simulink library "common_lib"  (R2023a)
settings: Solver=ode45  StartTime=0.0  StopTime=10.0  RelTol=1e-3
undefined symbols (not defined in the file): ACCEL_PRE_MULT, APDT_SrvcMgr_IRVHVDCSubFcnReq, C_C1GearNumbers, C_C1GearRatios, C_Calibration, C_DitherWaveform, C_GearOffset, C_GearRatioIn, C_GearRatioInverseOut, C_GearRatioOut, CLUTCH_INNER_LOOP_UPDATE_RATE, CONSTANT, DEGRADED_MODE_SIZE, Dem_EventStatusType, DiscIntNeverNeededParam, F_FAULT_ENUM, F_NOFAULT, F_OUTOFRANGE, F_RATELIMIT, FALSE, FMI14_SPECIAL_INSTRUCTIONS, FMI20_DATA_DRIFTED_HIGH, FMI21_DATA_DRIFTED_LOW, FMI29_RESERVED_FOR_SAE_ASSIGNMENT, FMI30_RESERVED_FOR_SAE_ASSIGNMENT, FMI31_CONDITION_EXISTS, FMI32_NO_FAULT, IC, k_accel, k_mean, MAX_UINT32, MEAN_PRE_MULT, NTriggers, QLTY_SIGNAL_FAILED, QLTY_SIGNAL_FULLY_FUNCTION, QLTY_SIGNAL_SUBSTITUTED_BY_1ST_CHOICE, QLTY_SIGNAL_SUBSTITUTED_BY_2ND_CHOICE, QLTY_SIGNAL_SUBSTITUTED_BY_3RD_CHOICE, QLTY_SIGNAL_SUBSTITUTED_BY_4TH_CHOICE, SAMPLE_TIME_100us, SAMPLETIME_10ms_Int, SATURATION_U16, simin, T_TestPoint, TF_FALSE, TF_TRUE, TimeStep, TRUE, WORKSPACE_UPDATE_RATE, ZERO, Zero
libraries: $bdroot x123, simulink x28, simulink_extras x4, MBD_EPS_Local_Blockset x4
(part 6 of 10)

== system common_lib/Diagnostics/DiagDbncCntrLite ==
  DiagFaultCntThresh : Inport
  DiagPassCntThresh : Inport  Port=2
  DiagFaultActive : Inport  Port=3
  DiagReset : Inport  Port=4
  diagHealEn : Inport  Port=5
  Constant1 : Constant  Value=int16(1)
  Constant2 : Constant  Value=int16(1)
  DiagDebounce_CCaller : CCaller  FunctionName=DiagDebounceLite  PortSpecificationStruct="%)30     .    :!    8    (     @         %    \"     D    !     0         %  0 \"0    $    _    07)G3F%M90  4&]R=$YA;64 4V-O<&4     26YD97@     5'EP90      4VEZ90      27-';&]B86P   X   !     !@    @    $          4    (     0   !     !         !     0    9&EA9T9A=6QT0V]U;G1E<@X   !     !@    @    $          4    (     0   !     !         !     0    9&EA9T9A=6QT0V]U;G1E<@X   !     !@    @    $     ...(+5283 chars)"
  Unit Delay : UnitDelay  SampleTime=-1  HasFrameUpgradeWarning=on
      settings: AttributesFormatString=%<InitialCondition>
  Unit Delay1 : UnitDelay  InitialCondition=int8(0)  SampleTime=-1  HasFrameUpgradeWarning=on
      settings: AttributesFormatString=%<InitialCondition>
  DiagCurrState : Outport  VectorParamsAs1DForOutWhenUnconnected=off
  wires:
  diagHealEn/1 -> DiagDebounce_CCaller/9
  Constant2/1 -> DiagDebounce_CCaller/8
  Constant1/1 -> DiagDebounce_CCaller/7
  DiagReset/1 -> DiagDebounce_CCaller/4
  DiagDebounce_CCaller/2 -> DiagCurrState/1, Unit Delay1/1
  DiagPassCntThresh/1 -> DiagDebounce_CCaller/6
  DiagFaultCntThresh/1 -> DiagDebounce_CCaller/5
  DiagFaultActive/1 -> DiagDebounce_CCaller/3
  Unit Delay/1 -> DiagDebounce_CCaller/1
  Unit Delay1/1 -> DiagDebounce_CCaller/2
  DiagDebounce_CCaller/1 -> Unit Delay/1

== system common_lib/Diagnostics/DiagFaultCounter ==
  diagFaultActive : Inport
  diagStartUpComp : Inport  Port=2
  diagReset : Inport  Port=3
  diagEnable : Inport  Port=4
  diagDbncEnab : Inport  Port=5
  diagFaultCntThresh : Inport  Port=6
  diagPassCntThresh : Inport  Port=7
  diagUpCnt : Inport  Port=8
  diagDnCnt : Inport  Port=9
  diagHealEn : Inport  Port=10
  DiagFaulCounter : Stateflow chart  TreatAsAtomicUnit=on
  diagFaultStatus : Outport  OutputWhenDisabled=reset  InitialOutput=Dem_EventStatusType.DEM_EVENT_STATUS_INIT  VectorParamsAs1DForOutWhenUnconnected=off
  wires:
  diagHealEn/1 -> DiagFaulCounter/10(diagHealEn)
  diagPassCntThresh/1 -> DiagFaulCounter/7(diagPassCntThresh)
  diagStartUpComp/1 -> DiagFaulCounter/2(diagStartUpComp)
  diagDbncEnab/1 -> DiagFaulCounter/5(diagDbncEnab)
  DiagFaulCounter/1(diagFaultStatus) -> diagFaultStatus/1
  diagEnable/1 -> DiagFaulCounter/4(diagEnable)
  diagDnCnt/1 -> DiagFaulCounter/9(diagDnCnt)
  diagUpCnt/1 -> DiagFaulCounter/8(diagUpCnt)
  diagReset/1 -> DiagFaulCounter/3(diagReset)
  diagFaultCntThresh/1 -> DiagFaulCounter/6(diagFaultCntThresh)
  diagFaultActive/1 -> DiagFaulCounter/1(diagFaultActive)

== system common_lib/Diagnostics/ExtractValue ==
  in : Inport  OutDataTypeStr=Bus: BO_InputSignal
  Bus Selector : BusSelector  OutputSignals=value,FMI
  value : Outport  VectorParamsAs1DForOutWhenUnconnected=off
  FMI : Outport  Port=2  VectorParamsAs1DForOutWhenUnconnected=off
  wires:
  Bus Selector/2 -> FMI/1  "<FMI>"
  in/1 -> Bus Selector/1
  Bus Selector/1 -> value/1  "<value>"

== system common_lib/Diagnostics/FMIUpdate ==
  UpdateFaultStatus : Inport
  FMI_In : Inport  Port=2
  FMI_UpdateValue : Inport  Port=3
  Constant2 : Constant  Value=FMI32_NO_FAULT  SampleTime=-1
  Relational Operator3 : RelationalOperator  Operator=~=  ZeroCross=off  InputSameDT=off
  Switch : Switch  Threshold=0.5  ZeroCross=off  SaturateOnIntegerOverflow=off  InputSameDT=off
  Switch1 : Switch  Threshold=0.5  ZeroCross=off  SaturateOnIntegerOverflow=off  InputSameDT=off
  FMI_Out : Outport  VectorParamsAs1DForOutWhenUnconnected=off
  wires:
  Switch1/1 -> FMI_Out/1
  FMI_In/1 -> Switch/3, Switch1/1, Relational Operator3/1
  Relational Operator3/1 -> Switch1/2
  Switch/1 -> Switch1/3
  FMI_UpdateValue/1 -> Switch/1
  UpdateFaultStatus/1 -> Switch/2
  Constant2/1 -> Relational Operator3/2

== system common_lib/Diagnostics/Fault Debounce Lv1 Boolean Input ==
  diagInput : Inport
  diagStartUpComp : Inport  Port=2
  diagUpCnt : Inport  Port=3
  diagDnCnt : Inport  Port=4
  diagFaultCntThresh : Inport  Port=5
  diagPassCntThresh : Inport  Port=6
  diagDbncEnab : Inport  Port=7
  diagReset : Inport  Port=8
  diagEnable : Inport  Port=9
  diagHealEn : Inport  Port=10
  diagPreestorageEn : Inport  Port=11
  diagJumpDownEn : Inport  Port=12
  Ccaller_DiagLv1 : $bdroot/Diagnostics/Ccaller_DiagLv1  SystemSampleTime=-1  VariantActivationTime=update diagram  Latency=0  AutoFrameSizeCalculation=off
  diagFaultStatus : Outport  OutputWhenDisabled=reset  InitialOutput=Dem_EventStatusType.DEM_EVENT_STATUS_INIT  VectorParamsAs1DForOutWhenUnconnected=off
  diagPreestorageTrigger : Outport  Port=2  OutputWhenDisabled=reset  InitialOutput=Dem_EventStatusType.DEM_EVENT_STATUS_INIT  VectorParamsAs1DForOutWhenUnconnected=off
  wires:
  diagStartUpComp/1 -> Ccaller_DiagLv1/2
  diagReset/1 -> Ccaller_DiagLv1/3
  diagEnable/1 -> Ccaller_DiagLv1/4
  diagDbncEnab/1 -> Ccaller_DiagLv1/5
  diagFaultCntThresh/1 -> Ccaller_DiagLv1/6
  diagPassCntThresh/1 -> Ccaller_DiagLv1/7
  diagUpCnt/1 -> Ccaller_DiagLv1/8
  diagDnCnt/1 -> Ccaller_DiagLv1/9
  diagHealEn/1 -> Ccaller_DiagLv1/10
  diagPreestorageEn/1 -> Ccaller_DiagLv1/11
  diagJumpDownEn/1 -> Ccaller_DiagLv1/12
  Ccaller_DiagLv1/2 -> diagPreestorageTrigger/1
  Ccaller_DiagLv1/1 -> diagFaultStatus/1
  diagInput/1 -> Ccaller_DiagLv1/1

== system common_lib/Diagnostics/Fault Debounce Lv1 state Input ==
  diagInput : Inport
  diagStartUpComp : Inport  Port=2
  diagMaxVal : Inport  Port=3
  diagMinVal : Inport  Port=4
  diagUpCnt : Inport  Port=5
  diagDnCnt : Inport  Port=6
  diagFaultCntThresh : Inport  Port=7
  diagPassCntThresh : Inport  Port=8
  diagDbncEnab : Inport  Port=9
  diagReset : Inport  Port=10
  diagEnable : Inport  Port=11
  diagHealEn : Inport  Port=12
  diagPreestorageEn : Inport  Port=13
  diagJumpDownEn : Inport  Port=14
  Ccaller_DiagLv1 : $bdroot/Diagnostics/Ccaller_DiagLv1  SystemSampleTime=-1  VariantActivationTime=update diagram  Latency=0  AutoFrameSizeCalculation=off
  OR : Logic  Operator=OR  AllPortsSameDT=off  OutDataTypeStr=boolean
  Relational Operator : RelationalOperator  OutDataTypeStr=boolean  ZeroCross=off  InputSameDT=off
  Relational Operator1 : RelationalOperator  Operator=<=  OutDataTypeStr=boolean  ZeroCross=off  InputSameDT=off
  diagFaultStatus : Outport  OutputWhenDisabled=reset  InitialOutput=Dem_EventStatusType.DEM_EVENT_STATUS_INIT  VectorParamsAs1DForOutWhenUnconnected=off
  diagPreestorageTrigger : Outport  Port=2  OutputWhenDisabled=reset  InitialOutput=Dem_EventStatusType.DEM_EVENT_STATUS_INIT  VectorParamsAs1DForOutWhenUnconnected=off
  wires:
  diagMaxVal/1 -> Relational Operator/2
  diagReset/1 -> Ccaller_DiagLv1/3
  diagDnCnt/1 -> Ccaller_DiagLv1/9
  diagFaultCntThresh/1 -> Ccaller_DiagLv1/6
  diagPassCntThresh/1 -> Ccaller_DiagLv1/7
  diagUpCnt/1 -> Ccaller_DiagLv1/8
  Relational Operator/1 -> OR/1
  diagStartUpComp/1 -> Ccaller_DiagLv1/2
  diagDbncEnab/1 -> Ccaller_DiagLv1/5
  diagInput/1 -> Relational Operator/1, Relational Operator1/1
  diagHealEn/1 -> Ccaller_DiagLv1/10
  diagMinVal/1 -> Relational Operator1/2
  OR/1 -> Ccaller_DiagLv1/1
  Relational Operator1/1 -> OR/2
  diagEnable/1 -> Ccaller_DiagLv1/4
  diagPreestorageEn/1 -> Ccaller_DiagLv1/11
  diagJumpDownEn/1 -> Ccaller_DiagLv1/12
  Ccaller_DiagLv1/1 -> diagFaultStatus/1
  Ccaller_DiagLv1/2 -> diagPreestorageTrigger/1

== system common_lib/Diagnostics/FaultStatusUpdate ==
  FMI_In : Inport
  DriftLow : Inport  Port=2
  DriftHigh : Inport  Port=3
  SpecialInstructions : Inport  Port=4
  ConditionExists : Inport  Port=5
  DriftLowSubReqest : Inport  Port=6
  DriftLowSubReqest1 : Inport  Port=7
  Constant : Constant  Value=FMI14_SPECIAL_INSTRUCTIONS  SampleTime=-1
  Constant1 : Constant  Value=FMI21_DATA_DRIFTED_LOW  SampleTime=-1
  Constant2 : Constant  Value=FMI20_DATA_DRIFTED_HIGH  SampleTime=-1
  Constant3 : Constant  Value=FMI29_RESERVED_FOR_SAE_ASSIGNMENT  SampleTime=-1
  Constant4 : Constant  Value=FMI32_NO_FAULT  SampleTime=-1
  Constant5 : Constant  Value=FMI30_RESERVED_FOR_SAE_ASSIGNMENT  SampleTime=-1
  Constant6 : Constant  Value=FMI31_CONDITION_EXISTS  SampleTime=-1
  Relational Operator3 : RelationalOperator  Operator=~=  ZeroCross=off  InputSameDT=off
  Switch{,1..6} (7 alike) : Switch  Threshold=0.5  ZeroCross=off  SaturateOnIntegerOverflow=off  InputSameDT=off
  FMI_Out : Outport  VectorParamsAs1DForOutWhenUnconnected=off
  wires:
  Switch1/1 -> FMI_Out/1
  Constant4/1 -> Relational Operator3/2
  Switch/1 -> Switch1/3
  Relational Operator3/1 -> Switch1/2
  FMI_In/1 -> Relational Operator3/1, Switch1/1, Switch6/3
  Switch2/1 -> Switch/3
  Switch3/1 -> Switch2/3
  Switch4/1 -> Switch3/3
  DriftLow/1 -> Switch/2
  Constant1/1 -> Switch/1
  Constant2/1 -> Switch2/1
  DriftHigh/1 -> Switch2/2
  Constant/1 -> Switch3/1
  SpecialInstructions/1 -> Switch3/2
  Constant6/1 -> Switch4/1
  ConditionExists/1 -> Switch4/2
  Constant3/1 -> Switch5/1
  DriftLowSubReqest/1 -> Switch5/2
  Constant5/1 -> Switch6/1
  DriftLowSubReqest1/1 -> Switch6/2
  Switch6/1 -> Switch5/3
  Switch5/1 -> Switch4/3

== system common_lib/Diagnostics/Heal Enable Cnt With Reset ==
  Diag_FltSts : Inport
  Mode_Req : Inport  Port=2
  Diag_TogLim_C : Inport  Port=3
  Accumulator : UnitDelay  SampleTime=-1  HasFrameUpgradeWarning=on
      settings: AttributesFormatString=ic=%<X0>
  ActFltSts : RelationalOperator  Operator===  ZeroCross=off  InputSameDT=off
  CntrCnd : Switch  Criteria=u2 ~= 0  Threshold=0.5  ZeroCross=off  SaturateOnIntegerOverflow=off  InputSameDT=off
      settings: AttributesFormatString=%<Criteria>
  DIAG_FLTD : Constant  OutDataTypeStr=uint8  SampleTime=-1
  DIAG_FLTD1 : Constant  OutDataTypeStr=uint8  SampleTime=-1
  EdgeDetection : Logic  AllPortsSameDT=off
  HealEnaCnd : RelationalOperator  Operator=<=  OutDataTypeStr=boolean  ZeroCross=off  InputSameDT=off
  HealEnaCnd_Old : UnitDelay  SampleTime=-1  HasFrameUpgradeWarning=on
      settings: AttributesFormatString=ic=%<X0>
  IncrCond : Logic  AllPortsSameDT=off
  OldFltSts : RelationalOperator  Operator=~=  ZeroCross=off  InputSameDT=off
  PM_STANDBY : Constant  Value=0  OutDataTypeStr=uint8  SampleTime=-1
  Plus_One : Constant  OutDataTypeStr=uint8  SampleTime=-1
  Plus_Zero : Constant  Value=0  OutDataTypeStr=uint8  SampleTime=-1
  ResetCond : RelationalOperator  Operator===  ZeroCross=off  InputSameDT=off
  Reset_Value : Constant  Value=0  OutDataTypeStr=uint8  SampleTime=-1
  RstCnd : Switch  Criteria=u2 ~= 0  Threshold=0.5  ZeroCross=off  SaturateOnIntegerOverflow=off  InputSameDT=off
      settings: AttributesFormatString=%<Criteria>
  Sum2 : Sum  Inputs=|++
  Unit Delay1 : UnitDelay  InitialCondition=FALSE  SampleTime=-1  HasFrameUpgradeWarning=on
      settings: AttributesFormatString=ic=%<X0>
  Diag_HealEna : Outport  VectorParamsAs1DForOutWhenUnconnected=off
  wires:
  RstCnd/1 -> Accumulator/1, HealEnaCnd/1
  Sum2/1 -> RstCnd/3
  ResetCond/1 -> RstCnd/2
  Diag_TogLim_C/1 -> HealEnaCnd/2
  Plus_Zero/1 -> CntrCnd/3
  OldFltSts/1 -> EdgeDetection/2
  Unit Delay1/1 -> OldFltSts/1
  HealEnaCnd_Old/1 -> IncrCond/2
  HealEnaCnd/1 -> Diag_HealEna/1, HealEnaCnd_Old/1
  Plus_One/1 -> CntrCnd/1
  CntrCnd/1 -> Sum2/1
  IncrCond/1 -> CntrCnd/2
  Diag_FltSts/1 -> Unit Delay1/1, ActFltSts/1
  Reset_Value/1 -> RstCnd/1
  ActFltSts/1 -> EdgeDetection/1
  DIAG_FLTD1/1 -> OldFltSts/2
  DIAG_FLTD/1 -> ActFltSts/2
  Accumulator/1 -> Sum2/2
  Mode_Req/1 -> ResetCond/1
  PM_STANDBY/1 -> ResetCond/2
  EdgeDetection/1 -> IncrCond/1

== system common_lib/Diagnostics/KeepAlive ==
  State : Inport  OutDataTypeStr=boolean  PortDimensions=1
  A : Inport  Port=2  PortDimensions=1
  B : Inport  Port=3  PortDimensions=1
  Delay : UnitDelay  InitialCondition=false  SampleTime=-1  HasFrameUpgradeWarning=on
  Logical Operator : Logic  Operator=OR  AllPortsSameDT=off  OutDataTypeStr=boolean
  RelOp : RelationalOperator  Operator===  OutDataTypeStr=boolean
  Enable : Outport  OutDataTypeStr=boolean  PortDimensions=1  VectorParamsAs1DForOutWhenUnconnected=off
  Rel : Outport  Port=2  OutDataTypeStr=boolean  PortDimensions=1  VectorParamsAs1DForOutWhenUnconnected=off
  wires:
  RelOp/1 -> Logical Operator/2, Rel/1
  Logical Operator/1 -> Enable/1
  B/1 -> RelOp/2
  Delay/1 -> Logical Operator/1
  State/1 -> Delay/1
  A/1 -> RelOp/1

== system common_lib/Diagnostics/LogicBasedActivation ==
  note: Logic Based Activation
  Enable : Inport  OutDataTypeStr=boolean  PortDimensions=1
  DMToAdd : Inport  Port=2  OutDataTypeStr=uint32  PortDimensions=DM_SIZE
  Add : Inport  Port=3  OutDataTypeStr=boolean  PortDimensions=1
  DMPackedData_in : Inport  Port=4  OutDataTypeStr=uint32  PortDimensions=DM_SIZE
  Bitwise Operator : simulink/Logic and Bit Operations/Bitwise Operator  logicop=OR  UseBitMask=off  NumInputPorts=2  BitMask=bin2dec('11011001')  BitMaskRealWorld=Stored Integer
  Logical Operator1 : Logic  AllPortsSameDT=off
  Switch3 : Switch  Threshold=0.5  ZeroCross=off  SaturateOnIntegerOverflow=off  InputSameDT=off
  DMPackedData_out : Outport  OutDataTypeStr=uint32  PortDimensions=DM_SIZE  VectorParamsAs1DForOutWhenUnconnected=off
  wires:
  Switch3/1 -> DMPackedData_out/1
  Bitwise Operator/1 -> Switch3/1
  DMToAdd/1 -> Bitwise Operator/1
  DMPackedData_in/1 -> Bitwise Operator/2, Switch3/3
  Logical Operator1/1 -> Switch3/2
  Enable/1 -> Logical Operator1/1
  Add/1 -> Logical Operator1/2

== system common_lib/Diagnostics/LogicBasedDeactivation ==
  note: Logic Based Deactivation
  Enable : Inport  OutDataTypeStr=boolean  PortDimensions=1
  DMToRemove : Inport  Port=2  OutDataTypeStr=uint32  PortDimensions=DM_SIZE
  Remove : Inport  Port=3  OutDataTypeStr=boolean  PortDimensions=1
  DMPackedData_in : Inport  Port=4  OutDataTypeStr=uint32  PortDimensions=DM_SIZE
  Bitwise Operator : simulink/Logic and Bit Operations/Bitwise Operator  logicop=AND  UseBitMask=off  NumInputPorts=2  BitMask=bin2dec('11011001')  BitMaskRealWorld=Stored Integer
  Bitwise Operator1 : simulink/Logic and Bit Operations/Bitwise Operator  logicop=NOT  UseBitMask=off  BitMask=bin2dec('11011001')  BitMaskRealWorld=Stored Integer
  Logical Operator1 : Logic  AllPortsSameDT=off
  Switch3 : Switch  Threshold=0.5  ZeroCross=off  SaturateOnIntegerOverflow=off  InputSameDT=off
  DMPackedData_out : Outport  OutDataTypeStr=uint32  PortDimensions=DM_SIZE  VectorParamsAs1DForOutWhenUnconnected=off
  wires:
  Remove/1 -> Logical Operator1/2
  Enable/1 -> Logical Operator1/1
  Logical Operator1/1 -> Switch3/2
  DMPackedData_in/1 -> Switch3/3, Bitwise Operator/2
  DMToRemove/1 -> Bitwise Operator1/1
  Bitwise Operator/1 -> Switch3/1
  Switch3/1 -> DMPackedData_out/1
  Bitwise Operator1/1 -> Bitwise Operator/1

== system common_lib/Diagnostics/OOR Fault Detect Enum ==
  note: Common Library::Diagnostics::Out of Range Fault Detection with Enable for Enum
  in : Inport
  Enable : Inport  Port=2
  Logical Operator1 : Logic  Operator=NOT  AllPortsSameDT=off  OutDataTypeStr=boolean
  Switch : Switch  Criteria=u2 ~= 0  InputSameDT=off
  detect fault : Subsystem
  false1 : Constant  Value=FALSE  OutDataTypeStr=boolean
  out : Outport  VectorParamsAs1DForOutWhenUnconnected=off
  fault? : Outport  Port=2  VectorParamsAs1DForOutWhenUnconnected=off
  wires:
  Enable/1 -> Logical Operator1/1, detect fault/Enable
  Switch/1 -> fault?/1
  false1/1 -> Switch/1
  detect fault/1(fault set) -> Switch/3
  in/1 -> out/1, detect fault/1(In1)
  Logical Operator1/1 -> Switch/2

== system common_lib/Diagnostics/OOR Fault Detection ==
  note: Common Library::Diagnostics::Out of Range Fault Detection with Enable
  in : Inport
  Enable : Inport  Port=2
  Logical Operator3 : Logic  Operator=NOT  AllPortsSameDT=off  OutDataTypeStr=boolean
  Switch : Switch  Criteria=u2 ~= 0  InputSameDT=off
  detect fault : Subsystem
  false : Constant  Value=FALSE  OutDataTypeStr=boolean
  out : Outport  VectorParamsAs1DForOutWhenUnconnected=off
  fault? : Outport  Port=2  VectorParamsAs1DForOutWhenUnconnected=off
  wires:
  in/1 -> out/1, detect fault/1(In1)
  Logical Operator3/1 -> Switch/2
  detect fault/1(fault set) -> Switch/3
  false/1 -> Switch/1
  Switch/1 -> fault?/1
  Enable/1 -> Logical Operator3/1, detect fault/Enable

== system common_lib/Diagnostics/SetFMI ==
  FMI_in : Inport  OutDataTypeStr=uint8  PortDimensions=1
  Active1 : Inport  Port=2  OutDataTypeStr=boolean  PortDimensions=1
  Active2 : Inport  Port=3  OutDataTypeStr=boolean  PortDimensions=1
  Active3 : Inport  Port=4  OutDataTypeStr=boolean  PortDimensions=1
  Active4 : Inport  Port=5  OutDataTypeStr=boolean  PortDimensions=1
  Active5 : Inport  Port=6  OutDataTypeStr=boolean  PortDimensions=1
  Active6 : Inport  Port=7  OutDataTypeStr=boolean  PortDimensions=1
  Active7 : Inport  Port=8  OutDataTypeStr=boolean  PortDimensions=1
  Constant : Constant  Value=PRIORITY_1_FMI
  Constant1 : Constant  Value=PRIORITY_2_FMI
  Constant2 : Constant  Value=PRIORITY_3_FMI
  Constant3 : Constant  Value=PRIORITY_4_FMI
  Constant4 : Constant  Value=PRIORITY_5_FMI
  Constant5 : Constant  Value=PRIORITY_6_FMI
  Constant6 : Constant  Value=PRIORITY_7_FMI
  IF_ELSE_LADDER : Subsystem  TreatAsAtomicUnit=on
      settings: RTWSystemCode=Inline
  FMI_out : Outport  VectorParamsAs1DForOutWhenUnconnected=off
  wires:
  IF_ELSE_LADDER/1(FMI_out) -> FMI_out/1
  Active7/1 -> IF_ELSE_LADDER/8(Active7)
  Active6/1 -> IF_ELSE_LADDER/7(Active6)
  Active5/1 -> IF_ELSE_LADDER/6(Active5)
  Active4/1 -> IF_ELSE_LADDER/5(Active4)
  Active3/1 -> IF_ELSE_LADDER/4(Active3)
  Active2/1 -> IF_ELSE_LADDER/3(Active2)
  Active1/1 -> IF_ELSE_LADDER/2(Active1)
  FMI_in/1 -> IF_ELSE_LADDER/1(FMI_in)
  Constant6/1 -> IF_ELSE_LADDER/15(FMI_7)
  Constant5/1 -> IF_ELSE_LADDER/14(FMI_6)
  Constant4/1 -> IF_ELSE_LADDER/13(FMI_5)
  Constant3/1 -> IF_ELSE_LADDER/12(FMI_4)
  Constant2/1 -> IF_ELSE_LADDER/11(FMI_3)
  Constant1/1 -> IF_ELSE_LADDER/10(FMI_2)
  Constant/1 -> IF_ELSE_LADDER/9(FMI_1)

== system common_lib/Diagnostics/SignalSubstitution ==
  Signal_in : Inport  OutDataTypeStr=single  PortDimensions=1
  SignalFaulted : Inport  Port=2  OutDataTypeStr=boolean  PortDimensions=1
  FirstChoiceSubstitute : Inport  Port=3  OutDataTypeStr=single  PortDimensions=1
  FirstChoiceFaulted : Inport  Port=4  OutDataTypeStr=boolean  PortDimensions=1
  SecondChoiceSubstitute : Inport  Port=5  OutDataTypeStr=single  PortDimensions=1
  SecondChoiceFaulted : Inport  Port=6  OutDataTypeStr=boolean  PortDimensions=1
  ThirdChoiceSubstitute : Inport  Port=7  OutDataTypeStr=single  PortDimensions=1
  ThirdChoiceFaulted : Inport  Port=8  OutDataTypeStr=boolean  PortDimensions=1
  FourthChoiceSubstitute : Inport  Port=9  OutDataTypeStr=single  PortDimensions=1
  FourthChoiceFaulted : Inport  Port=10  OutDataTypeStr=boolean  PortDimensions=1
  FailedValue : Inport  Port=11  OutDataTypeStr=single  PortDimensions=1
  If : If  NumInputs=5  IfExpression=~u1  ElseIfExpressions=~u2, ~u3, ~u4, ~u5
  If Action Subsystem : Subsystem  TreatAsAtomicUnit=on
  If Action Subsystem1 : Subsystem  TreatAsAtomicUnit=on
  If Action Subsystem2 : Subsystem  TreatAsAtomicUnit=on
  If Action Subsystem3 : Subsystem  TreatAsAtomicUnit=on
  If Action Subsystem4 : Subsystem  TreatAsAtomicUnit=on
  If Action Subsystem5 : Subsystem  TreatAsAtomicUnit=on
  Merge : Merge  Inputs=6
  Merge1 : Merge  Inputs=6
  Signal_out : Outport  OutDataTypeStr=single  PortDimensions=1  VectorParamsAs1DForOutWhenUnconnected=off
  Qlty : Outport  Port=2  OutDataTypeStr=uint8  PortDimensions=1  VectorParamsAs1DForOutWhenUnconnected=off
  wires:
  If Action Subsystem2/2(Qlty) -> Merge1/3
  If Action Subsystem2/1(Signal) -> Merge/3
  If Action Subsystem1/2(Qlty) -> Merge1/2
  If Action Subsystem3/1(Signal) -> Merge/4
  Merge/1 -> Signal_out/1
  If Action Subsystem4/2(Qlty) -> Merge1/5
  If Action Subsystem/1(Signal) -> Merge/1
  If Action Subsystem4/1(Signal) -> Merge/5
  If Action Subsystem5/1(Signal) -> Merge/6
  If Action Subsystem1/1(Signal) -> Merge/2
  If Action Subsystem3/2(Qlty) -> Merge1/4
  If Action Subsystem/2(Qlty) -> Merge1/1
  If Action Subsystem5/2(Qlty) -> Merge1/6
  Merge1/1 -> Qlty/1
  If/3 -> If Action Subsystem2/Action
  Signal_in/1 -> If Action Subsystem/1(NoSubstitute)
  SecondChoiceSubstitute/1 -> If Action Subsystem2/1(SecondChoice)
  If/1 -> If Action Subsystem/Action
  FirstChoiceFaulted/1 -> If/2
  If/2 -> If Action Subsystem1/Action
  SecondChoiceFaulted/1 -> If/3
  FourthChoiceFaulted/1 -> If/5
  FirstChoiceSubstitute/1 -> If Action Subsystem1/1(FirstChoice)
  If/4 -> If Action Subsystem3/Action
  ThirdChoiceFaulted/1 -> If/4
  FailedValue/1 -> If Action Subsystem5/1(FailedValue)
  If/5 -> If Action Subsystem4/Action
  If/6 -> If Action Subsystem5/Action
  SignalFaulted/1 -> If/1
  FourthChoiceSubstitute/1 -> If Action Subsystem4/1(FourthChoice)
  ThirdChoiceSubstitute/1 -> If Action Subsystem3/1(ThirdChoice)

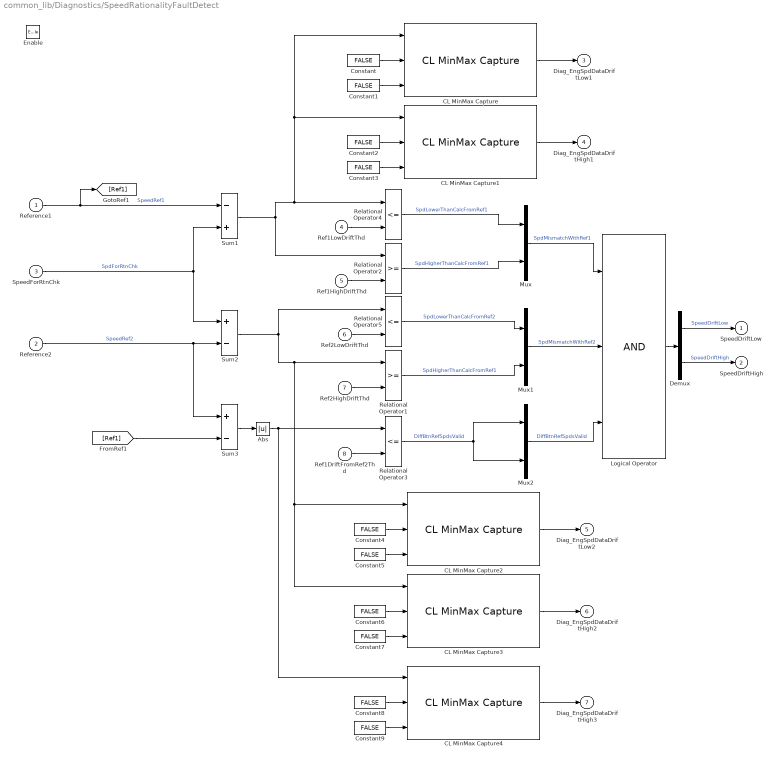
== system common_lib/Diagnostics/SpeedRationalityFaultDetect ==
  Reference1 : Inport
  Reference2 : Inport  Port=2
  SpeedForRtnChk : Inport  Port=3
  Ref1LowDriftThd : Inport  Port=4
  Ref1HighDriftThd : Inport  Port=5
  Ref2LowDriftThd : Inport  Port=6
  Ref2HighDriftThd : Inport  Port=7
  Ref1DriftFromRef2Thd : Inport  Port=8
  Enable : EnablePort  ZeroCross=off
  Abs : Abs  ZeroCross=off  SaturateOnIntegerOverflow=off
  CL MinMax Capture : $bdroot/Diag/CL MinMax Capture  CaptureType=Min  InDataType=single
  CL MinMax Capture1 : $bdroot/Diag/CL MinMax Capture  CaptureType=Max  InDataType=single
  CL MinMax Capture2 : $bdroot/Diag/CL MinMax Capture  CaptureType=Min  InDataType=single
  CL MinMax Capture3 : $bdroot/Diag/CL MinMax Capture  CaptureType=Max  InDataType=single
  CL MinMax Capture4 : $bdroot/Diag/CL MinMax Capture  CaptureType=Max  InDataType=single
  Constant{,1..9} (10 alike) : Constant  Value=FALSE  SampleTime=-1
  Demux : Demux  Outputs=2
  Logical Operator : Logic  Inputs=3  AllPortsSameDT=off
  Mux : Mux  Inputs=2
  Mux1 : Mux  Inputs=2
  Mux2 : Mux  Inputs=2
  Relational Operator1 : RelationalOperator  ZeroCross=off  InputSameDT=off
  Relational Operator2 : RelationalOperator  ZeroCross=off  InputSameDT=off
  Relational Operator3 : RelationalOperator  Operator=<=  ZeroCross=off  InputSameDT=off
  Relational Operator4 : RelationalOperator  Operator=<=  ZeroCross=off  InputSameDT=off
  Relational Operator5 : RelationalOperator  Operator=<=  ZeroCross=off  InputSameDT=off
  Sum1 : Sum  Inputs=-+
  Sum2 : Sum  Inputs=+-
  Sum3 : Sum  Inputs=+-
  SpeedDriftLow : Outport  OutputWhenDisabled=reset  InitialOutput=[0]  VectorParamsAs1DForOutWhenUnconnected=off
  SpeedDriftHigh : Outport  Port=2  OutputWhenDisabled=reset  InitialOutput=[0]  VectorParamsAs1DForOutWhenUnconnected=off
  Diag_EngSpdDataDriftLow1 : Outport  Port=3  InitialOutput=[0]  VectorParamsAs1DForOutWhenUnconnected=off
  Diag_EngSpdDataDriftHigh1 : Outport  Port=4  InitialOutput=[0]  VectorParamsAs1DForOutWhenUnconnected=off
  Diag_EngSpdDataDriftLow2 : Outport  Port=5  InitialOutput=[0]  VectorParamsAs1DForOutWhenUnconnected=off
  Diag_EngSpdDataDriftHigh2 : Outport  Port=6  InitialOutput=[0]  VectorParamsAs1DForOutWhenUnconnected=off
  Diag_EngSpdDataDriftHigh3 : Outport  Port=7  InitialOutput=[0]  VectorParamsAs1DForOutWhenUnconnected=off
  wires:
  Constant9/1 -> CL MinMax Capture4/3
  Constant8/1 -> CL MinMax Capture4/2
  CL MinMax Capture4/1 -> Diag_EngSpdDataDriftHigh3/1
  CL MinMax Capture3/1 -> Diag_EngSpdDataDriftHigh2/1
  CL MinMax Capture2/1 -> Diag_EngSpdDataDriftLow2/1
  Constant7/1 -> CL MinMax Capture3/3
  Constant6/1 -> CL MinMax Capture3/2
  Constant5/1 -> CL MinMax Capture2/3
  Constant4/1 -> CL MinMax Capture2/2
  CL MinMax Capture1/1 -> Diag_EngSpdDataDriftHigh1/1
  CL MinMax Capture/1 -> Diag_EngSpdDataDriftLow1/1
  Constant3/1 -> CL MinMax Capture1/3
  Constant2/1 -> CL MinMax Capture1/2
  Constant1/1 -> CL MinMax Capture/3
  Constant/1 -> CL MinMax Capture/2
  Reference2/1 -> Sum3/1, Sum2/2  "SpeedRef2"
  Reference1/1 -> [Ref1], Sum1/1  "SpeedRef1"
  Ref2HighDriftThd/1 -> Relational Operator1/2
  Ref1HighDriftThd/1 -> Relational Operator2/2
  Logical Operator/1 -> Demux/1
  Demux/2 -> SpeedDriftHigh/1  "SpeedDriftHigh"
  Demux/1 -> SpeedDriftLow/1  "SpeedDriftLow"
  Mux2/1 -> Logical Operator/3  "DiffBtnRefSpdsValid"
  Mux1/1 -> Logical Operator/2  "SpdMismatchWithRef2"
  Mux/1 -> Logical Operator/1  "SpdMismatchWithRef1"
  Relational Operator1/1 -> Mux1/2  "SpdHigherThanCalcFromRef1"
  Relational Operator5/1 -> Mux1/1  "SpdLowerThanCalcFromRef2"
  Relational Operator4/1 -> Mux/1  "SpdLowerThanCalcFromRef1"
  Sum3/1 -> Abs/1
  Ref2LowDriftThd/1 -> Relational Operator5/2
  Ref1LowDriftThd/1 -> Relational Operator4/2
  Ref1DriftFromRef2Thd/1 -> Relational Operator3/2
  Abs/1 -> CL MinMax Capture4/1, Relational Operator3/1
  Sum2/1 -> Relational Operator5/1, Relational Operator1/1, CL MinMax Capture3/1, CL MinMax Capture2/1
  [Ref1] -> Sum3/2
  SpeedForRtnChk/1 -> Sum2/1, Sum1/2  "SpdForRtnChk"
  Relational Operator2/1 -> Mux/2  "SpdHigherThanCalcFromRef1"
  Sum1/1 -> Relational Operator2/1, Relational Operator4/1, CL MinMax Capture/1, CL MinMax Capture1/1
  Relational Operator3/1 -> Mux2/2, Mux2/1  "DiffBtnRefSpdsValid"

== system common_lib/Diagnostics/ToRWSignal ==
  in : Inport
  FMI : Inport  Port=2
  Bus Creator2 : BusCreator  Inputs=2  OutDataTypeStr=Bus: BO_InputSignal
  Data Type Conversion1 : DataTypeConversion  OutDataTypeStr=single  SaturateOnIntegerOverflow=off  RndMeth=Floor
  Data Type Conversion2 : DataTypeConversion  OutDataTypeStr=uint8  SaturateOnIntegerOverflow=off  RndMeth=Floor
  out : Outport  VectorParamsAs1DForOutWhenUnconnected=off
  wires:
  FMI/1 -> Data Type Conversion2/1
  Data Type Conversion2/1 -> Bus Creator2/2  "FMI"
  Data Type Conversion1/1 -> Bus Creator2/1  "value"
  in/1 -> Data Type Conversion1/1
  Bus Creator2/1 -> out/1

== system common_lib/Documentation/EatonLogo ==

== system common_lib/Documentation/LegalNoticeEaton ==

== system common_lib/Documentation/RequirementLinks ==
  DocBlock : simulink/Model-Wide Utilities/DocBlock  DocumentType=Text
      content=|
      | REQ_1234

== system common_lib/Documentation/SubsystemPath ==

== system common_lib/Fltrs/Fltr ==
  note: Common Library::Filters::Filter
  input : Inport
  tau : Inport  Port=2
  Constant : Constant  Value=single(0)  SampleTime=-1
  Constant1 : Constant  Value=false  SampleTime=-1
  Constant2 : Constant  Value=false  SampleTime=-1
  Data Type Conversion : DataTypeConversion  OutDataTypeStr=single  SaturateOnIntegerOverflow=off  RndMeth=Floor
  Data Type Conversion1 : DataTypeConversion  OutDataTypeStr=single  SaturateOnIntegerOverflow=off  RndMeth=Floor
  FilterCoreLogic1 : $bdroot/Fltrs/Fltr_wRO/FilterCoreLogic  SystemSampleTime=-1  VariantActivationTime=update diagram  Latency=0  AutoFrameSizeCalculation=off
  Signal Conversion : SignalConversion  ConversionOutput=Contiguous copy  OverrideOpt=on
  output : Outport  VectorParamsAs1DForOutWhenUnconnected=off
  wires:
  input/1 -> Data Type Conversion/1
  tau/1 -> Data Type Conversion1/1
  Signal Conversion/1 -> output/1
  FilterCoreLogic1/1 -> Signal Conversion/1
  Constant/1 -> FilterCoreLogic1/3
  Constant1/1 -> FilterCoreLogic1/4
  Constant2/1 -> FilterCoreLogic1/5
  Data Type Conversion/1 -> FilterCoreLogic1/1
  Data Type Conversion1/1 -> FilterCoreLogic1/2

== system common_lib/Fltrs/Fltr_wR ==
  note: Common Library::Filters::Filter with Reset
  note: This is a simple 1st order filter block with reset.
      |
      |     if reset is true (1) then output=ic
      |    otherwise output = previous output + (input - previous output) * T/tau
  input : Inport
  tau : Inport  Port=2
  ic : Inport  Port=3
  reset? : Inport  Port=4  OutDataTypeStr=boolean
  Constant : Constant  Value=false  SampleTime=-1
  Data Type Conversion : DataTypeConversion  OutDataTypeStr=single  SaturateOnIntegerOverflow=off  RndMeth=Floor
  Data Type Conversion1 : DataTypeConversion  OutDataTypeStr=single  SaturateOnIntegerOverflow=off  RndMeth=Floor
  Data Type Conversion2 : DataTypeConversion  OutDataTypeStr=single  SaturateOnIntegerOverflow=off  RndMeth=Floor
  Data Type Conversion3 : DataTypeConversion  OutDataTypeStr=boolean  SaturateOnIntegerOverflow=off  RndMeth=Floor
  FilterCoreLogic1 : $bdroot/Fltrs/Fltr_wRO/FilterCoreLogic  SystemSampleTime=-1  VariantActivationTime=update diagram  Latency=0  AutoFrameSizeCalculation=off
  Signal Conversion : SignalConversion  ConversionOutput=Contiguous copy  OverrideOpt=on
  output : Outport  VectorParamsAs1DForOutWhenUnconnected=off
  wires:
  ic/1 -> Data Type Conversion2/1
  reset?/1 -> Data Type Conversion3/1
  input/1 -> Data Type Conversion/1
  tau/1 -> Data Type Conversion1/1
  FilterCoreLogic1/1 -> Signal Conversion/1
  Signal Conversion/1 -> output/1
  Constant/1 -> FilterCoreLogic1/5
  Data Type Conversion/1 -> FilterCoreLogic1/1
  Data Type Conversion1/1 -> FilterCoreLogic1/2
  Data Type Conversion2/1 -> FilterCoreLogic1/3
  Data Type Conversion3/1 -> FilterCoreLogic1/4

== system common_lib/Fltrs/Fltr_wRO ==
  note: This is a simple 1st order filter block with reset and override.
      |
      |      If override is true (1) then output=override_value
      |      If       reset is true (1) then output=input
      |    otherwise output = previous output + (input - previous output) * T/tau
  note: Common Library::Filters::Filter with Reset and Override
  input : Inport
  tau : Inport  Port=2
  override_value : Inport  Port=3
  override? : Inport  Port=4  OutDataTypeStr=boolean
  reset? : Inport  Port=5  OutDataTypeStr=boolean
  Data Type Conversion : DataTypeConversion  OutDataTypeStr=single  SaturateOnIntegerOverflow=off  RndMeth=Floor
  Data Type Conversion1 : DataTypeConversion  OutDataTypeStr=single  SaturateOnIntegerOverflow=off  RndMeth=Floor
  Data Type Conversion2 : DataTypeConversion  OutDataTypeStr=single  SaturateOnIntegerOverflow=off  RndMeth=Floor
  Data Type Conversion3 : DataTypeConversion  OutDataTypeStr=boolean  SaturateOnIntegerOverflow=off  RndMeth=Floor
  Data Type Conversion4 : DataTypeConversion  OutDataTypeStr=boolean  SaturateOnIntegerOverflow=off  RndMeth=Floor
  FilterCoreLogic : Subsystem  TreatAsAtomicUnit=on  RTWFcnName=FLTR
      settings: RTWFcnNameOpts=User specified  RTWFileNameOpts=Use function name
  Signal Conversion : SignalConversion  ConversionOutput=Contiguous copy  OverrideOpt=on
  output : Outport  VectorParamsAs1DForOutWhenUnconnected=off
  wires:
  FilterCoreLogic/1(output) -> Signal Conversion/1
  tau/1 -> Data Type Conversion1/1
  input/1 -> Data Type Conversion/1
  Signal Conversion/1 -> output/1
  reset?/1 -> Data Type Conversion4/1
  override_value/1 -> Data Type Conversion2/1
  override?/1 -> Data Type Conversion3/1
  Data Type Conversion/1 -> FilterCoreLogic/1(input)
  Data Type Conversion1/1 -> FilterCoreLogic/2(tau)
  Data Type Conversion2/1 -> FilterCoreLogic/3(override_value)
  Data Type Conversion3/1 -> FilterCoreLogic/4(override?)
  Data Type Conversion4/1 -> FilterCoreLogic/5(reset?)

== system common_lib/Fltrs/Fltr_wROExtInitCond ==
  note: This is a simple 1st order filter block with reset and override.
      |
      |      If override is true (1) then output=override_value
      |      If       reset is true (1) then output=input
      |    otherwise output = previous output + (input - previous output) * T/tau
  note: Common Library::Filters::Filter with Reset and Override
  input : Inport
  tau : Inport  Port=2
  init_cond : Inport  Port=3  OutDataTypeStr=single
  reset : Inport  Port=4  OutDataTypeStr=boolean
  override : Inport  Port=5  OutDataTypeStr=boolean
  override_value : Inport  Port=6
  Constant1 : Constant  Value=Ts
  Data Type Conversion{,1..2,5..6} (5 alike) : DataTypeConversion  OutDataTypeStr=single  SaturateOnIntegerOverflow=off  RndMeth=Floor
  Data Type Conversion3 : DataTypeConversion  OutDataTypeStr=boolean  SaturateOnIntegerOverflow=off  RndMeth=Floor
  Data Type Conversion4 : DataTypeConversion  OutDataTypeStr=boolean  SaturateOnIntegerOverflow=off  RndMeth=Floor
  FilterCoreLogic : Subsystem  RTWFcnName=FLTR
      settings: RTWFcnNameOpts=User specified  RTWFileNameOpts=Use function name
  Signal Conversion : SignalConversion  ConversionOutput=Contiguous copy  OverrideOpt=on
  output : Outport  VectorParamsAs1DForOutWhenUnconnected=off
  wires:
  init_cond/1 -> Data Type Conversion6/1
  FilterCoreLogic/1(output) -> Signal Conversion/1
  tau/1 -> Data Type Conversion1/1
  input/1 -> Data Type Conversion/1
  Signal Conversion/1 -> output/1
  reset/1 -> Data Type Conversion4/1
  override_value/1 -> Data Type Conversion2/1
  override/1 -> Data Type Conversion3/1
  Data Type Conversion3/1 -> FilterCoreLogic/6(override)
  Data Type Conversion2/1 -> FilterCoreLogic/7(override_value)
  Data Type Conversion/1 -> FilterCoreLogic/1(input)
  Data Type Conversion4/1 -> FilterCoreLogic/5(reset)
  Data Type Conversion1/1 -> FilterCoreLogic/2(tau)
  Data Type Conversion6/1 -> FilterCoreLogic/3(init_cond)
  Constant1/1 -> Data Type Conversion5/1
  Data Type Conversion5/1 -> FilterCoreLogic/4(task_rate)

== system common_lib/Fltrs/Int16FIR ==
  u : Inport  OutDataTypeStr=int16
  Accum : Subsystem  TreatAsAtomicUnit=on
  Buffer : simulink/Discrete/Tapped Delay  vinit=0.0  samptime=-1  NumDelays=2*N  DelayOrder=Newest  includeCurrent=off
  Constant : Constant  Value=MEAN_PRE_MULT
  Constant1 : Constant  Value=ACCEL_PRE_MULT
  Constant2 : Constant  Value=int32(N)
  Constant3 : Constant  Value=int32(2^(k_accel-1))
  Constant4 : Constant  Value=int32(2^(k_mean-1))
  Data Type Conversion : DataTypeConversion  OutDataTypeStr=int16  RndMeth=Floor
  Data Type Conversion1 : DataTypeConversion  OutDataTypeStr=int16  SaturateOnIntegerOverflow=off  RndMeth=Floor
  Data Type Conversion2 : DataTypeConversion  OutDataTypeStr=int32  SaturateOnIntegerOverflow=off  RndMeth=Floor
  Data Type Conversion3 : DataTypeConversion  OutDataTypeStr=int32  SaturateOnIntegerOverflow=off  RndMeth=Floor
  Data Type Conversion4 : DataTypeConversion  OutDataTypeStr=int32  SaturateOnIntegerOverflow=off  RndMeth=Floor
  Product : Product  OutDataTypeStr=int32
  Product1 : Product  OutDataTypeStr=int32
  Product2 : Product  OutDataTypeStr=int32
  Selector : Selector  IndexMode=Zero-based  InputPortWidth=2*N  IndexOptions=Index vector (dialog)  Indices=N-1  OutputSizes=1
  Selector1 : Selector  IndexMode=Zero-based  InputPortWidth=2*N  IndexOptions=Index vector (dialog)  Indices=2*N-1  OutputSizes=1
  Shift Arithmetic : ArithShift  BitShiftNumber=k_mean
  Shift Arithmetic1 : ArithShift  BitShiftNumber=k_accel
  Sum{,1,4..6} (5 alike) : Sum  Inputs=|++
  Sum2 : Sum  Inputs=++|
  Sum3 : Sum  Inputs=|+-
  Mean : Outport  VectorParamsAs1DForOutWhenUnconnected=off
  Accel : Outport  Port=2  VectorParamsAs1DForOutWhenUnconnected=off
  wires:
  Constant4/1 -> Sum6/2
  Sum6/1 -> Shift Arithmetic/1
  Constant3/1 -> Sum5/2
  Sum5/1 -> Shift Arithmetic1/1
  Product2/1 -> Sum4/2
  Sum4/1 -> Product1/1
  Constant2/1 -> Product2/2
  Sum3/1 -> Product2/1
  Data Type Conversion4/1 -> Sum2/1, Sum3/1
  Sum2/1 -> Sum1/2
  Data Type Conversion3/1 -> Sum2/2, Sum3/2
  Data Type Conversion2/1 -> Sum1/1
  Selector1/1 -> Data Type Conversion3/1
  u/1 -> Buffer/1, Data Type Conversion4/1
  Data Type Conversion/1 -> Accel/1
  Sum/1 -> Product/1
  Product/1 -> Sum6/1
  Constant/1 -> Product/2
  Shift Arithmetic/1 -> Data Type Conversion1/1
  Constant1/1 -> Product1/2
  Product1/1 -> Sum5/1
  Buffer/1 -> Accum/1(Buf), Selector/1, Selector1/1
  Shift Arithmetic1/1 -> Data Type Conversion/1
  Accum/1(Accel_Accum) -> Sum4/1
  Selector/1 -> Data Type Conversion2/1
  Data Type Conversion1/1 -> Mean/1
  Sum1/1 -> Sum/2
  Accum/2(Mean_Accum) -> Sum/1

== system common_lib/Fltrs/Inv_Fltr ==
  note: This is the inverse of a simple 1st order filter block
  note: Common Library::Filters::Inverse Filter
  input : Inport
  tau : Inport  Port=2
  Constant1 : Constant  Value=TimeStep
  Constant2 : Constant  Value=false
  Data Type Conversion : DataTypeConversion  OutDataTypeStr=single  SaturateOnIntegerOverflow=off  RndMeth=Floor
  Product : Product  Inputs=*/  InputSameDT=on  OutDataTypeStr=Inherit: Same as first input
  Product1 : Product  Inputs=**  InputSameDT=on  OutDataTypeStr=Inherit: Same as first input
  Sum : Sum  Inputs=-+|  InputSameDT=on  OutDataTypeStr=Inherit: Same as first input
  Sum1 : Sum  Inputs=++|  InputSameDT=on  OutDataTypeStr=Inherit: Same as first input
  Switch1 : Switch  Threshold=0.5  ZeroCross=off  SaturateOnIntegerOverflow=off
  Unit Delay1 : UnitDelay  InitialCondition=Zero  SampleTime=-1  HasFrameUpgradeWarning=on
      settings: AttributesFormatString=ic=%<X0>
  Unit Delay2 : UnitDelay  InitialCondition=true  SampleTime=-1  HasFrameUpgradeWarning=on
      settings: AttributesFormatString=ic=%<X0>
  output : Outport  VectorParamsAs1DForOutWhenUnconnected=off
  wires:
  Constant1/1 -> Data Type Conversion/1
  Data Type Conversion/1 -> Product/2
  Unit Delay2/1 -> Switch1/2
  Constant2/1 -> Unit Delay2/1
  Switch1/1 -> Sum1/1, Sum/1
  Unit Delay1/1 -> Switch1/3
  Sum1/1 -> output/1
  Product1/1 -> Sum1/2
  Product/1 -> Product1/2
  Sum/1 -> Product1/1
  tau/1 -> Product/1
  input/1 -> Unit Delay1/1, Switch1/1, Sum/2

== system common_lib/Fltrs/Inv_RpdFltr ==
  note: u(k) = y(k-1) + ( y(k) - y(k-1) )/fc
  note: Common Library::Filters::Inverse Rapid Filtering
  input : Inport
  fltr_cnst : Inport  Port=2
  Constant1 : Constant  Value=single(eps)
  Constant3 : Constant  Value=false
  MinMax : MinMax  Function=max  Inputs=2  InputSameDT=on  SaturateOnIntegerOverflow=on  ZeroCross=off
  Product : Product  Inputs=*/  InputSameDT=on  OutDataTypeStr=Inherit: Same as first input
  Sum : Sum  Inputs=|+-  InputSameDT=on  OutDataTypeStr=Inherit: Same as first input
  Sum1 : Sum  Inputs=|++  InputSameDT=on  OutDataTypeStr=Inherit: Same as first input
  Switch2 : Switch  Threshold=0.5  ZeroCross=off  SaturateOnIntegerOverflow=off
  Unit Delay3 : UnitDelay  InitialCondition=Zero  SampleTime=-1  HasFrameUpgradeWarning=on
      settings: AttributesFormatString=ic=%<X0>
  Unit Delay4 : UnitDelay  InitialCondition=true  SampleTime=-1  HasFrameUpgradeWarning=on
      settings: AttributesFormatString=ic=%<X0>
  output : Outport  VectorParamsAs1DForOutWhenUnconnected=off
  wires:
  Switch2/1 -> Sum/2
  Unit Delay4/1 -> Switch2/2
  Constant3/1 -> Unit Delay4/1
  Unit Delay3/1 -> Switch2/3
  fltr_cnst/1 -> MinMax/2
  MinMax/1 -> Product/2
  Constant1/1 -> MinMax/1
  input/1 -> Switch2/1, Unit Delay3/1, Sum/1
  Sum/1 -> Product/1
  Product/1 -> Sum1/1
  Sum1/1 -> output/1

== system common_lib/Fltrs/Lookup_wFltr ==
  input : Inport
  x-axis_vector : Inport  Port=2
  y-axis_vector : Inport  Port=3
  override? : Inport  Port=4
  override_value : Inport  Port=5
  filter_enable? : Inport  Port=6
  tau : Inport  Port=7
  ic : Inport  Port=8
  2D Lookup : $bdroot/Tbl/2D Lookup
  Fltr_wROExtInitCond : $bdroot/Fltrs/Fltr_wROExtInitCond  TimeStep=Ts
  NOT : Logic  Operator=NOT  AllPortsSameDT=off  OutDataTypeStr=boolean
  output : Outport  VectorParamsAs1DForOutWhenUnconnected=off
  wires:
  Fltr_wROExtInitCond/1 -> output/1
  input/1 -> 2D Lookup/1
  y-axis_vector/1 -> 2D Lookup/3
  x-axis_vector/1 -> 2D Lookup/2
  2D Lookup/1 -> Fltr_wROExtInitCond/1
  filter_enable?/1 -> NOT/1
  NOT/1 -> Fltr_wROExtInitCond/4
  tau/1 -> Fltr_wROExtInitCond/2
  ic/1 -> Fltr_wROExtInitCond/3
  override?/1 -> Fltr_wROExtInitCond/5
  override_value/1 -> Fltr_wROExtInitCond/6

== system common_lib/Fltrs/Rpd_Fltr ==
  note: Common Library::Filters::Rapid Filter
  note: Y(k) = FC * ( X(k) - Y(k-1)) + Y(k-1)
  input : Inport
  fltr_cnst : Inport  Port=2
  Product : Product  Inputs=**  InputSameDT=on  OutDataTypeStr=Inherit: Same as first input
  Sum : Sum  Inputs=|+-  InputSameDT=on  OutDataTypeStr=Inherit: Same as first input
  Sum1 : Sum  Inputs=|++  InputSameDT=on  OutDataTypeStr=Inherit: Same as first input
  Unit Delay : UnitDelay  InitialCondition=IC  SampleTime=-1  HasFrameUpgradeWarning=on
  output : Outport  VectorParamsAs1DForOutWhenUnconnected=off
  wires:
  Sum/1 -> Product/1
  input/1 -> Sum/1
  Unit Delay/1 -> Sum/2, Sum1/2
  fltr_cnst/1 -> Product/2
  Product/1 -> Sum1/1
  Sum1/1 -> output/1, Unit Delay/1

== system common_lib/Fltrs/Scaling_wFltr ==
  input : Inport
  res : Inport  Port=2
  offset : Inport  Port=3
  override : Inport  Port=4
  override_value : Inport  Port=5
  filter_enable : Inport  Port=6
  tau : Inport  Port=7
  init_cond : Inport  Port=8
  Add : Sum
  Fltr_wROExtInitCond : $bdroot/Fltrs/Fltr_wROExtInitCond  TimeStep=Ts
  NOT : Logic  Operator=NOT  AllPortsSameDT=off  OutDataTypeStr=boolean
  Product : Product
  output : Outport  VectorParamsAs1DForOutWhenUnconnected=off
  wires:
  Fltr_wROExtInitCond/1 -> output/1
  res/1 -> Product/2
  Add/1 -> Fltr_wROExtInitCond/1
  offset/1 -> Add/2
  input/1 -> Product/1
  Product/1 -> Add/1
  NOT/1 -> Fltr_wROExtInitCond/4
  filter_enable/1 -> NOT/1
  tau/1 -> Fltr_wROExtInitCond/2
  init_cond/1 -> Fltr_wROExtInitCond/3
  override/1 -> Fltr_wROExtInitCond/5
  override_value/1 -> Fltr_wROExtInitCond/6

== system common_lib/Fuzzy/Fuzzy Implication ==
  THEN : Inport
  Product : Product  RndMeth=Zero
  Select : BusSelector  OutputSignals=HighUpshiftPoint  OutputAsBus=on
  OUTPUT : Outport  VectorParamsAs1DForOutWhenUnconnected=off
  wires:
  THEN/1 -> Product/1
  [ShiftPoint] -> Select/1
  Select/1 -> Product/2
  Product/1 -> OUTPUT/1

== system common_lib/Fuzzy/Fuzzy Intersection ==
  IF : Inport
  MinMax : MinMax  Inputs=2
  OR : Sum  Inputs=+
  Select : BusSelector  OutputSignals=Demand.value
  Sum : Sum  Inputs=|+-
  THEN : Outport  VectorParamsAs1DForOutWhenUnconnected=off
  ELSE : Outport  Port=2  VectorParamsAs1DForOutWhenUnconnected=off
  wires:
  [DataBus] -> Select/1
  OR/1 -> MinMax/2
  MinMax/1 -> Sum/2, THEN/1
  Sum/1 -> ELSE/1
  IF/1 -> Sum/1, MinMax/1
  Select/1 -> OR/1  "<value>"

== system common_lib/Fuzzy/Fuzzy Membership Function ==
  note: Triangle Membership Function
  note: This switch is initializing
      | a vector of zeros equal in
      | length to the breakpoints.
  u : Inport
  brkpts : Inport  Port=2
  Assignment : Assignment  IndexMode=Zero-based  IndexOptions=Index vector (port)  Indices=1  OutputSizes=1
  Assignment1 : Assignment  IndexMode=Zero-based  IndexOptions=Index vector (port)  Indices=1  OutputSizes=1
  Constant2 : Constant  Value=single(0)
  Constant3 : Constant  Value=single(1)
  Constant5 : Constant  Value=true
  Constant6 : Constant  Value=uint32(1)
  Prelookup : PreLookup  BreakpointsDataSource=Input port  BreakpointsData=[10:10:110]  FractionDataTypeStr=single
      settings: InputPortMap=u0,p1
  Sum : Sum  Inputs=|+-
  Sum1 : Sum  Inputs=|++
  Switch : Switch  Threshold=0.5  SaturateOnIntegerOverflow=off
  Outport : Outport  VectorParamsAs1DForOutWhenUnconnected=off
  wires:
  Constant6/1 -> Sum1/2
  u/1 -> Prelookup/1
  Assignment1/1 -> Outport/1
  brkpts/1 -> Prelookup/2, Switch/3
  Constant5/1 -> Switch/2
  Constant2/1 -> Switch/1
  Switch/1 -> Assignment/1
  Constant3/1 -> Sum/1
  Prelookup/1 -> Sum1/1, Assignment/3
  Sum1/1 -> Assignment1/3
  Assignment/1 -> Assignment1/1
  Sum/1 -> Assignment/2
  Prelookup/2 -> Sum/2, Assignment1/2
